simulink model "Tarea"  (R2015a)
settings: Solver=ode45  StartTime=0.0  StopTime=6  RelTol=1e-3
settings Model: Creator=Jesus  LastModifiedBy=Jesus

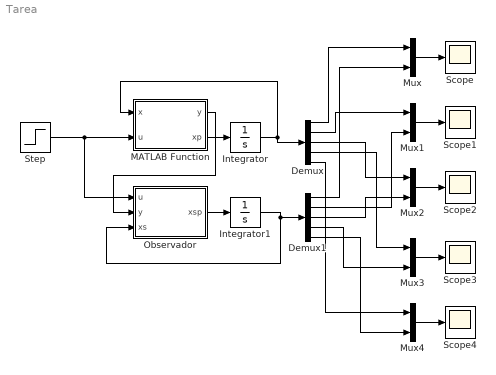
== system Tarea ==
  Demux : Demux  Outputs=5
  Demux1 : Demux  Outputs=5
  Integrator : Integrator  InitialCondition=[0 0 0 0 0]
  Integrator1 : Integrator  InitialCondition="[8  5 6 7 3]"
  MATLAB Function : MATLAB Function  TreatAsAtomicUnit=on
  Mux{,1..4} (5 alike) : Mux  Inputs=2
  Observador : MATLAB Function  TreatAsAtomicUnit=on
  Scope{,1..4} (5 alike) : Scope
      Scope2 settings: SaveName=ScopeData2
      Scope3 settings: SaveName=ScopeData3
      Scope4 settings: SaveName=ScopeData4
  Step : Step  SampleTime=0
  wires:
  MATLAB Function/2(xp) -> Integrator/1
  Step/1 -> Observador/1(u), MATLAB Function/2(u)
  Observador/1(xsp) -> Integrator1/1
  Integrator1/1 -> Demux1/1, Observador/3(xs)
  Integrator/1 -> Demux/1, MATLAB Function/1(x)
  Demux/1 -> Mux/1
  Demux1/1 -> Mux/2
  Demux/2 -> Mux1/1
  Demux1/2 -> Mux1/2
  Demux/3 -> Mux2/1
  Demux1/3 -> Mux2/2
  Demux/4 -> Mux3/1
  Demux1/4 -> Mux3/2
  Demux/5 -> Mux4/1
  Demux1/5 -> Mux4/2
  Mux/1 -> Scope/1
  Mux1/1 -> Scope1/1
  Mux2/1 -> Scope2/1
  Mux3/1 -> Scope3/1
  Mux4/1 -> Scope4/1
  MATLAB Function/1(y) -> Observador/2(y)

== matlab function Tarea/Observador ==
  data: u input; y input; xs input; xsp output
function xsp  = fcn(u,y,xs)
%#codegen
L=[10 -32 -71 32 -1]';
A=[0 -1 0 0 -4;0 0 1 0 1;0 1 0 0 2;-2 1 0 -2 4;0 0 0 0 -2];
B=[0 1 0 0 0]';
C=[1 0 0 0 0];
xsp=A*xs+B*u+L*(y-C*xs);

== matlab function Tarea/MATLAB Function ==
  data: x input; u input; y output; xp output
function [y, xp] = fcn(x,u)
%#codegen
A=[0 -1 0 0 -4;0 0 1 0 1;0 1 0 0 2;-2 1 0 -2 4;0 0 0 0 -2];
B=[0 1 0 0 0]';
C=[1 0 0 0 0];
xp=A*x+B*u;
y = C*x;
